simulink model "pixhawk_position"  (R2016b)
settings: Solver=FixedStepAuto  StartTime=0.0  StopTime=inf  FixedStep=0.01  RelTol=1e-3
PreLoadFcn:
  | load('bus_mavlink_att_pos_mocap_t.mat');
  | load('bus_mavlink_attitude_t.mat');
  | load('bus_mavlink_heartbeat_t.mat');
  | load('bus_mavlink_raw_imu_t.mat');
  | load('bus_mavlink_set_attitude_target_t.mat');
  | load('bus_mavlink_set_mode_t.mat');
  | load('bus_mavlink_set_position_target_local_ned_t.mat');
  | load('bus_mavlink_vicon_2q_t.mat');
libraries: dspnetwork x3, etargetslib x1, aerolibanimutils x1
settings Model: Creator=Admin  LastModifiedBy=luminghua

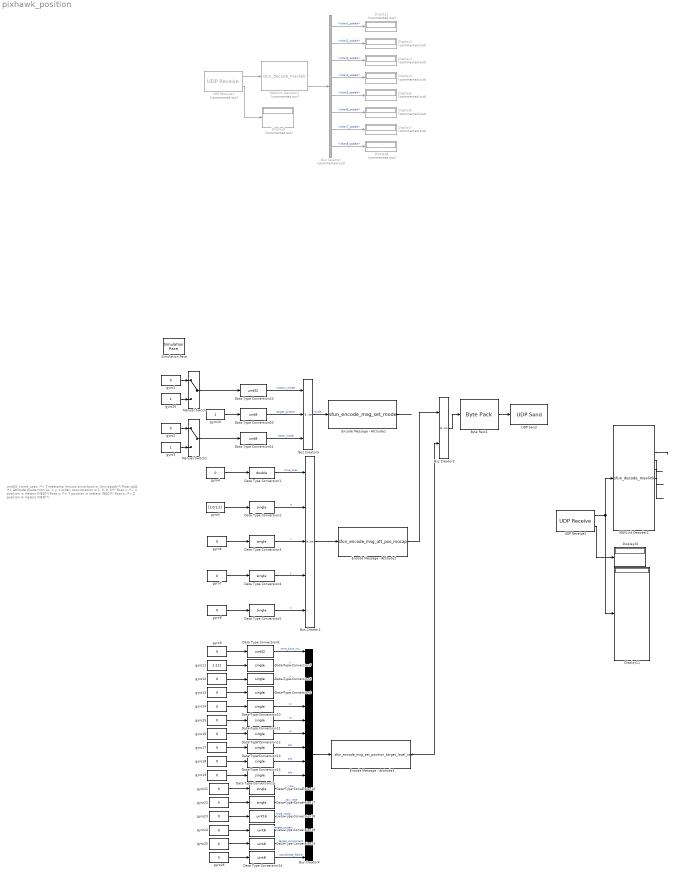
== system pixhawk_position ==
  note: uint64_t time_usec; /*< Timestamp (micros since boot or Unix epoch)*/
      |  float q[4]; /*< Attitude quaternion (w, x, y, z order, zero-rotation is 1, 0, 0, 0)*/
      |  float x; /*< X position in meters (NED)*/
      |  float y; /*< Y position in meters (NED)*/
      |  float z; /*< Z position in meters (NED)*/
  Bus Creator1 : BusCreator  Inputs=5  OutDataTypeStr=Bus: mavlink_att_pos_mocap_t
  Bus Creator2 : BusCreator  Inputs=2
  Bus Creator3 : BusCreator  Inputs=3  OutDataTypeStr=Bus: mavlink_set_mode_t
  Bus Creator4 : BusCreator  Inputs=16  OutDataTypeStr=Bus: mavlink_set_position_target_local_ned_t
  Bus Selector : BusSelector  Commented=on  OutputSignals=chan1_scaled,chan2_scaled,chan3_scaled,chan4_scaled,chan5_scaled,chan6_scaled,chan7_scaled,chan8_scaled
  Byte Pack1 : etargetslib/Byte Pack  datatypes={'uint8'}  byteAlign=1
  Data Type Conversion1 : DataTypeConversion  OutDataTypeStr=double
  Data Type Conversion{2..5,7..17} (15 alike) : DataTypeConversion  OutDataTypeStr=single
  Data Type Conversion18 : DataTypeConversion  OutDataTypeStr=uint16
  Data Type Conversion{19..21,23..24} (5 alike) : DataTypeConversion  OutDataTypeStr=uint8
  Data Type Conversion22 : DataTypeConversion  OutDataTypeStr=uint32
  Data Type Conversion6 : DataTypeConversion  OutDataTypeStr=uint32
  Display{1..9} (9 alike) : Display  Commented=on
  Display10 : Display
  Display11 : Display
  Encode Message - Attitude1 : S-Function  FunctionName=sfun_encode_msg_set_mode  SFunctionDeploymentMode=off  EnableBusSupport=off
  Encode Message - Attitude2 : S-Function  FunctionName=sfun_encode_msg_att_pos_mocap  SFunctionDeploymentMode=off  EnableBusSupport=off
  Encode Message - Attitude3 : S-Function  FunctionName=sfun_encode_msg_set_position_target_local_ned  SFunctionDeploymentMode=off  EnableBusSupport=off
  MAVLink Decoder1 : S-Function  Commented=on  FunctionName=sfun_decode_mavlink  SFunctionDeploymentMode=off  EnableBusSupport=off
  MAVLink Decoder2 : S-Function  FunctionName=sfun_decode_mavlink  SFunctionDeploymentMode=off  EnableBusSupport=off
  Manual Switch : ManualSwitch
  Manual Switch1 : ManualSwitch
  Simulation Pace : aerolibanimutils/Simulation Pace  SimulationPace=0.1  SleepMode=MATLAB Thread  OutputPaceError=off  SampleTime=0.01
  UDP Receive1 : dspnetwork/UDP Receive  Commented=on  localURL='0.0.0.0'  localPort=9750  remoteURL='0.0.0.0'  remotePort=-1  recvBufferSize=8192  dims=263  signalDatatype=uint8  isVarSize=off  showBlockingTime=on  blockingTime=0  sampletime=0.01  blockPlatform=HOST
  UDP Receive2 : dspnetwork/UDP Receive  localURL='0.0.0.0'  localPort=14550  remoteURL='192.168.1.101'  remotePort=-1  recvBufferSize=8192  dims=263  signalDatatype=uint8  isVarSize=off  showBlockingTime=on  blockingTime=0  sampletime=0.01  blockPlatform=HOST
  UDP Send : dspnetwork/UDP Send  remoteURL='192.168.1.100'  remotePort=9750  localURL='0.0.0.0'  localPortSource=Automatically determine  localPort=-1  sampletime=-1  blockPlatform=HOST  separateLengthPort=0
  gyro{1..2,4,6..9,12..19,21..25} (20 alike) : Constant  Value=0  SampleTime=-1
  gyro10 : Constant  SampleTime=-1
  gyro11 : Constant  Value=1.111  SampleTime=-1
  gyro20 : Constant  SampleTime=-1
  gyro26 : Constant  Value=3  SampleTime=-1
  gyro3 : Constant  SampleTime=-1
  gyro5 : Constant  Value=[1;0;1;2]  SampleTime=-1
  wires:
  Bus Selector/1 -> Display1/1  "<chan1_scaled>"
  Bus Selector/2 -> Display2/1  "<chan2_scaled>"
  Bus Selector/3 -> Display3/1  "<chan3_scaled>"
  Bus Selector/4 -> Display4/1  "<chan4_scaled>"
  Bus Selector/5 -> Display5/1  "<chan5_scaled>"
  Bus Selector/6 -> Display6/1  "<chan6_scaled>"
  Bus Selector/7 -> Display7/1  "<chan7_scaled>"
  Bus Selector/8 -> Display8/1  "<chan8_scaled>"
  UDP Receive1/1 -> MAVLink Decoder1/1
  UDP Receive1/2 -> Display9/1
  Encode Message - Attitude1/1 -> ?
  Bus Creator3/1 -> Encode Message - Attitude1/1  "mode"
  gyro10/1 -> Data Type Conversion20/1
  Manual Switch1/1 -> Data Type Conversion21/1
  Data Type Conversion21/1 -> Bus Creator3/3  "base_mode"
  Data Type Conversion20/1 -> Bus Creator3/2  "target_system"
  Data Type Conversion22/1 -> Bus Creator3/1  "custom_mode"
  Byte Pack1/1 -> UDP Send/1
  gyro1/1 -> Manual Switch/1
  Manual Switch/1 -> Data Type Conversion22/1
  gyro20/1 -> Manual Switch/2
  gyro2/1 -> Manual Switch1/1
  gyro3/1 -> Manual Switch1/2
  MAVLink Decoder1/5 -> Bus Selector/1
  UDP Receive2/1 -> Display11/1, MAVLink Decoder2/1
  UDP Receive2/2 -> Display10/1
  Bus Creator1/1 -> Encode Message - Attitude2/1
  Data Type Conversion1/1 -> Bus Creator1/1  "time_usec"
  Data Type Conversion2/1 -> Bus Creator1/2  "q"
  Data Type Conversion3/1 -> Bus Creator1/3  "x"
  Data Type Conversion4/1 -> Bus Creator1/4  "y"
  Data Type Conversion5/1 -> Bus Creator1/5  "z"
  gyro4/1 -> Data Type Conversion1/1
  gyro5/1 -> Data Type Conversion2/1
  gyro6/1 -> Data Type Conversion3/1
  gyro7/1 -> Data Type Conversion4/1
  gyro8/1 -> Data Type Conversion5/1
  Encode Message - Attitude2/1 -> Bus Creator2/1
  MAVLink Decoder2/3 -> ?
  MAVLink Decoder2/4 -> ?
  MAVLink Decoder2/5 -> ?
  MAVLink Decoder2/6 -> ?
  Bus Creator2/1 -> Byte Pack1/1
  Bus Creator4/1 -> Encode Message - Attitude3/1
  Data Type Conversion6/1 -> Bus Creator4/1  "time_boot_ms"
  Data Type Conversion7/1 -> Bus Creator4/2  "x"
  Data Type Conversion8/1 -> Bus Creator4/3  "y"
  Data Type Conversion9/1 -> Bus Creator4/4  "z"
  Data Type Conversion10/1 -> Bus Creator4/5  "vx"
  Data Type Conversion11/1 -> Bus Creator4/6  "vy"
  Data Type Conversion12/1 -> Bus Creator4/7  "vz"
  Data Type Conversion13/1 -> Bus Creator4/8  "afx"
  Data Type Conversion14/1 -> Bus Creator4/9  "afy"
  Data Type Conversion15/1 -> Bus Creator4/10  "afz"
  Data Type Conversion16/1 -> Bus Creator4/11  "yaw"
  Data Type Conversion17/1 -> Bus Creator4/12  "yaw_rate"
  Data Type Conversion18/1 -> Bus Creator4/13  "type_mask"
  Data Type Conversion19/1 -> Bus Creator4/14  "target_system"
  Data Type Conversion23/1 -> Bus Creator4/15  "target_component"
  Data Type Conversion24/1 -> Bus Creator4/16  "coordinate_frame"
  gyro9/1 -> Data Type Conversion6/1
  gyro11/1 -> Data Type Conversion7/1
  gyro12/1 -> Data Type Conversion8/1
  gyro13/1 -> Data Type Conversion9/1
  gyro14/1 -> Data Type Conversion10/1
  gyro15/1 -> Data Type Conversion11/1
  gyro16/1 -> Data Type Conversion12/1
  gyro17/1 -> Data Type Conversion13/1
  gyro18/1 -> Data Type Conversion14/1
  gyro19/1 -> Data Type Conversion15/1
  gyro21/1 -> Data Type Conversion16/1
  gyro22/1 -> Data Type Conversion17/1
  gyro23/1 -> Data Type Conversion18/1
  gyro24/1 -> Data Type Conversion19/1
  gyro25/1 -> Data Type Conversion23/1
  gyro26/1 -> Data Type Conversion24/1
  Encode Message - Attitude3/1 -> Bus Creator2/2
